simulink model "frame"  (R2020a)
settings: Solver=FixedStepAuto  StartTime=0.0  StopTime=10  FixedStep=1/simVars.freq  RelTol=1e-3
undefined symbols (not defined in the file or in its folder): par, sigbuilder_block, simVars
libraries: simulink x6
settings Model: Creator=Matthias  LastModifiedBy=sihao
settings DataIOCC: ReturnWorkspaceOutputs=off
settings DebuggingCC: ArithmeticOperatorsInVariantConditions=warning
settings SFSimCC: CustomCodeUndefinedFunction=UseInterfaceOnly

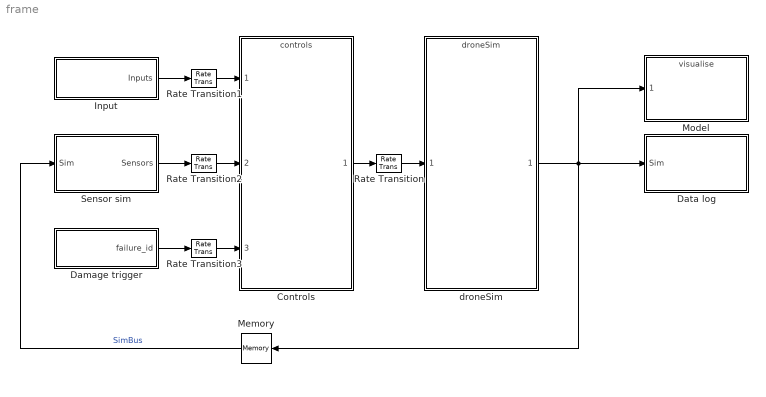
== system frame ==
  Controls : ModelReference  ModelNameDialog=controls  SimulationMode=Normal  ModelReferenceVersion=1.140
  Damage trigger : Subsystem
  Data log : Subsystem
  Input : Subsystem
  Memory : Memory
  Model : ModelReference  ModelNameDialog=visualise.slx  SimulationMode=Normal  ModelReferenceVersion=1.52
  Rate Transition : RateTransition  OutPortSampleTime=1/simVars.freq
  Rate Transition1 : RateTransition  OutPortSampleTime=1/par.freq
  Rate Transition2 : RateTransition  OutPortSampleTime=1/par.freq
  Rate Transition3 : RateTransition  OutPortSampleTime=1/par.freq
  Sensor sim : Subsystem
  droneSim : ModelReference  ModelNameDialog=droneSim  SimulationMode=Normal  ModelReferenceVersion=1.252
  wires:
  Input/1(Inputs) -> Rate Transition1/1
  Sensor sim/1(Sensors) -> Rate Transition2/1
  Memory/1 -> Sensor sim/1(Sim)  "SimBus"
  Rate Transition/1 -> droneSim/1
  Rate Transition1/1 -> Controls/1
  Rate Transition2/1 -> Controls/2
  Controls/1 -> Rate Transition/1
  droneSim/1 -> Model/1, Data log/1(Sim), Memory/1
  Damage trigger/1(failure_id) -> Rate Transition3/1
  Rate Transition3/1 -> Controls/3

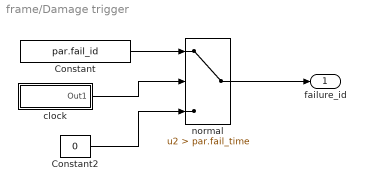
== system frame/Damage trigger ==
  Constant : Constant  Value=par.fail_id
  Constant2 : Constant  Value=0
  clock : Subsystem
  normal : Switch  Criteria=u2 > Threshold  Threshold=par.fail_time
  failure_id : Outport  VectorParamsAs1DForOutWhenUnconnected=off
  wires:
  Constant2/1 -> normal/3
  Constant/1 -> normal/1
  clock/1(Out1) -> normal/2
  normal/1 -> failure_id/1

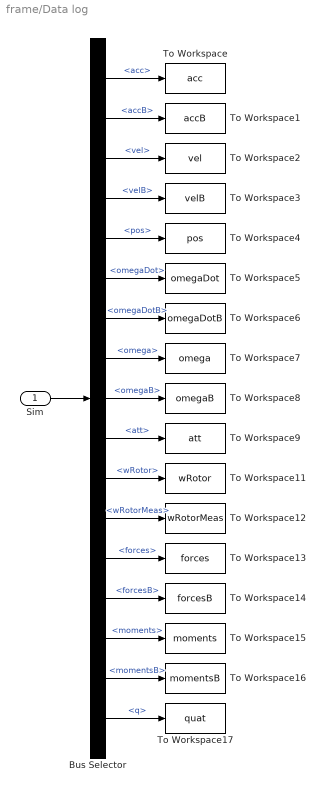
== system frame/Data log ==
  Sim : Inport
  Bus Selector : BusSelector  OutputSignals=acc,accB,vel,velB,pos,omegaDot,omegaDotB,omega,omegaB,att,wRotor,wRotorMeas,forces,forcesB,moments,momentsB,q
  To Workspace : ToWorkspace  VariableName=acc  SaveFormat=Timeseries  SampleTime=-1
  To Workspace1 : ToWorkspace  VariableName=accB  SaveFormat=Timeseries  SampleTime=-1
  To Workspace11 : ToWorkspace  VariableName=wRotor  SaveFormat=Timeseries  SampleTime=-1
  To Workspace12 : ToWorkspace  VariableName=wRotorMeas  SaveFormat=Timeseries  SampleTime=-1
  To Workspace13 : ToWorkspace  VariableName=forces  SaveFormat=Timeseries  SampleTime=-1
  To Workspace14 : ToWorkspace  VariableName=forcesB  SaveFormat=Timeseries  SampleTime=-1
  To Workspace15 : ToWorkspace  VariableName=moments  SaveFormat=Timeseries  SampleTime=-1
  To Workspace16 : ToWorkspace  VariableName=momentsB  SaveFormat=Timeseries  SampleTime=-1
  To Workspace17 : ToWorkspace  VariableName=quat  SaveFormat=Timeseries  SampleTime=-1
  To Workspace2 : ToWorkspace  VariableName=vel  SaveFormat=Timeseries  SampleTime=-1
  To Workspace3 : ToWorkspace  VariableName=velB  SaveFormat=Timeseries  SampleTime=-1
  To Workspace4 : ToWorkspace  VariableName=pos  SaveFormat=Timeseries  SampleTime=-1
  To Workspace5 : ToWorkspace  VariableName=omegaDot  SaveFormat=Timeseries  SampleTime=-1
  To Workspace6 : ToWorkspace  VariableName=omegaDotB  SaveFormat=Timeseries  SampleTime=-1
  To Workspace7 : ToWorkspace  VariableName=omega  SaveFormat=Timeseries  SampleTime=-1
  To Workspace8 : ToWorkspace  VariableName=omegaB  SaveFormat=Timeseries  SampleTime=-1
  To Workspace9 : ToWorkspace  VariableName=att  SaveFormat=Timeseries  SampleTime=-1
  wires:
  Sim/1 -> Bus Selector/1
  Bus Selector/1 -> To Workspace/1  "<acc>"
  Bus Selector/2 -> To Workspace1/1  "<accB>"
  Bus Selector/3 -> To Workspace2/1  "<vel>"
  Bus Selector/4 -> To Workspace3/1  "<velB>"
  Bus Selector/5 -> To Workspace4/1  "<pos>"
  Bus Selector/6 -> To Workspace5/1  "<omegaDot>"
  Bus Selector/7 -> To Workspace6/1  "<omegaDotB>"
  Bus Selector/8 -> To Workspace7/1  "<omega>"
  Bus Selector/9 -> To Workspace8/1  "<omegaB>"
  Bus Selector/10 -> To Workspace9/1  "<att>"
  Bus Selector/11 -> To Workspace11/1  "<wRotor>"
  Bus Selector/12 -> To Workspace12/1  "<wRotorMeas>"
  Bus Selector/13 -> To Workspace13/1  "<forces>"
  Bus Selector/14 -> To Workspace14/1  "<forcesB>"
  Bus Selector/15 -> To Workspace15/1  "<moments>"
  Bus Selector/16 -> To Workspace16/1  "<momentsB>"
  Bus Selector/17 -> To Workspace17/1  "<q>"

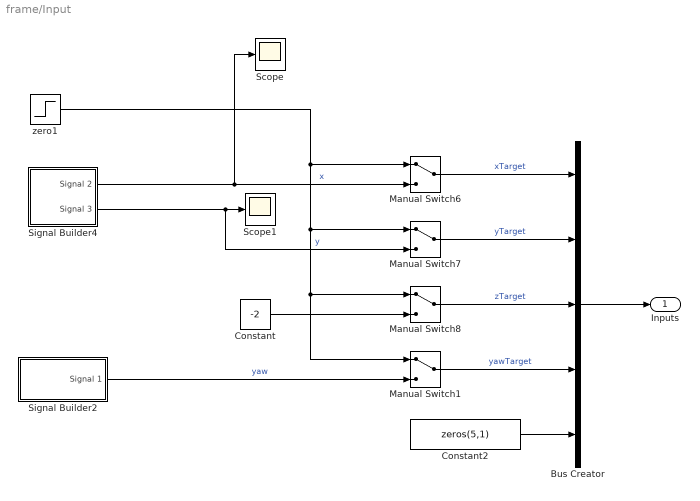
== system frame/Input ==
  Bus Creator : BusCreator  Inputs=5  OutDataTypeStr=Bus: inputsBus
  Constant : Constant  Value=-2
  Constant2 : Constant  Value=zeros(5,1)
  Manual Switch{1,6..8} (4 alike) : ManualSwitch
  Scope : Scope
  Scope1 : Scope
  Signal Builder2 : Subsystem  Tag=STV Subsys  LoadFcn=sigbuilder_block('load');  StartFcn=sigbuilder_block('start');  StopFcn=sigbuilder_block('stop');  ClipboardFcn=sigbuilder_block('clipboard');  mask(Sigbuilder block){tuvar=[0:10]}
      mask help: Simulink:masks:SigbuilderBlock_MD
      mask init:
      | if ~strcmp(get_param(bdroot(gcbh),'SimulationStatus'),'stopped') tuvar = sigbuilder_block('maskInit'); end
      settings: CopyFcn=sigbuilder_block('copy');  DeleteFcn=sigbuilder_block('delete');  ModelCloseFcn=sigbuilder_block('modelClose');  PreSaveFcn=sigbuilder_block('preSave');  PauseFcn=sigbuilder_block('pause');  ContinueFcn=sigbuilder_block('continue');  NameChangeFcn=sigbuilder_block('namechange');  OpenFcn=sigbuilder_block('open',[192.75 285.75 558 394.5 ]);  CloseFcn=sigbuilder_block('close');
      mask Display: plot(0, 0, 100, 100,[2, 2, 32, 32, 2], [68, 8, 8, 68, 68],[32, 2], [38, 38], [32, 19, 2],[53, 60, 44], [32, 17, 17, 2],[16, 16, 31, 31]);txt = getActiveGroup(gcbh);text(2, 100, txt,'verticalAlignment', 'top');
  Signal Builder4 : Subsystem  Tag=STV Subsys  LoadFcn=sigbuilder_block('load',[522.75 156 565.5 354 ]);  StartFcn=sigbuilder_block('start');  StopFcn=sigbuilder_block('stop');  ClipboardFcn=sigbuilder_block('clipboard');  mask(Sigbuilder block){tuvar=[0:10]}
      mask help: Simulink:masks:SigbuilderBlock_MD
      mask init:
      | if ~strcmp(get_param(bdroot(gcbh),'SimulationStatus'),'stopped') tuvar = sigbuilder_block('maskInit'); end
      settings: CopyFcn=sigbuilder_block('copy');  DeleteFcn=sigbuilder_block('delete');  ModelCloseFcn=sigbuilder_block('modelClose');  PreSaveFcn=sigbuilder_block('preSave');  PauseFcn=sigbuilder_block('pause');  ContinueFcn=sigbuilder_block('continue');  NameChangeFcn=sigbuilder_block('namechange');  OpenFcn=sigbuilder_block('open',[526.5 159.75 558 354 ]);  CloseFcn=sigbuilder_block('close');
      mask Display: plot(0, 0, 100, 100,[2, 2, 32, 32, 2], [68, 8, 8, 68, 68],[32, 2], [38, 38], [32, 19, 2],[53, 60, 44], [32, 17, 17, 2],[16, 16, 31, 31]);txt = getActiveGroup(gcbh);text(2, 100, txt,'verticalAlignment', 'top');
  zero1 : Step  Time=3  After=0  SampleTime=0
  Inputs : Outport  OutDataTypeStr=Bus: inputsBus  VectorParamsAs1DForOutWhenUnconnected=off
  wires:
  Bus Creator/1 -> Inputs/1
  Manual Switch1/1 -> Bus Creator/4  "yawTarget"
  Manual Switch8/1 -> Bus Creator/3  "zTarget"
  Constant/1 -> Manual Switch8/2
  Signal Builder4/2(Signal 3) -> Scope1/1, Manual Switch7/2  "y"
  Manual Switch6/1 -> Bus Creator/1  "xTarget"
  Manual Switch7/1 -> Bus Creator/2  "yTarget"
  Signal Builder4/1(Signal 2) -> Scope/1, Manual Switch6/2  "x"
  zero1/1 -> Manual Switch1/1, Manual Switch8/1, Manual Switch7/1, Manual Switch6/1
  Signal Builder2/1(Signal 1) -> Manual Switch1/2  "yaw"
  Constant2/1 -> Bus Creator/5

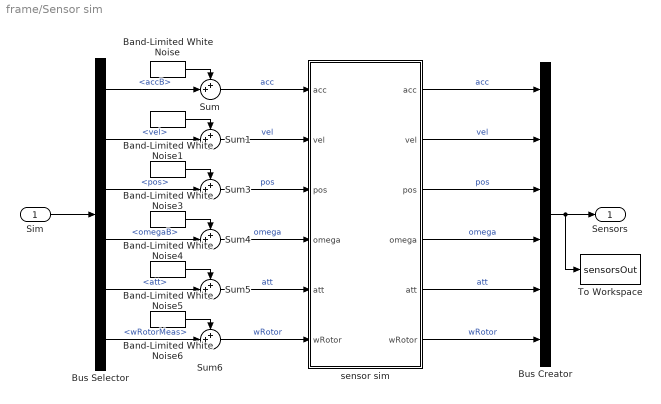
== system frame/Sensor sim ==
  Sim : Inport
  Band-Limited White Noise : simulink/Sources/Band-Limited White Noise  Cov=simVars.sensor.accNoise  Ts=1/par.freq  seed=[23341,23342,23343]
  Band-Limited White Noise1 : simulink/Sources/Band-Limited White Noise  Cov=simVars.sensor.velNoise  Ts=1/par.freq  seed=[23344,23345,23346]
  Band-Limited White Noise3 : simulink/Sources/Band-Limited White Noise  Cov=simVars.sensor.posNoise  Ts=1/par.freq  seed=[23347,23348,23349]
  Band-Limited White Noise4 : simulink/Sources/Band-Limited White Noise  Cov=simVars.sensor.omegaNoise  Ts=1/par.freq  seed=[23350,23351,23352]
  Band-Limited White Noise5 : simulink/Sources/Band-Limited White Noise  Cov=simVars.sensor.attNoise  Ts=1/par.freq  seed=[23353,23354,23355]
  Band-Limited White Noise6 : simulink/Sources/Band-Limited White Noise  Cov=simVars.sensor.wRotorNoise  Ts=1/par.freq  seed=[23356,23357,23358,23359]
  Bus Creator : BusCreator  Inputs=6  OutDataTypeStr=Bus: sensorsBus
      settings: InheritFromInputs=off
  Bus Selector : BusSelector  OutputSignals=accB,vel,pos,omegaB,att,wRotorMeas
  Sum{,1,3..6} (6 alike) : Sum  Inputs=++|
  To Workspace : ToWorkspace  VariableName=sensorsOut  SaveFormat=Timeseries  SampleTime=-1
  sensor sim : MATLAB Function  TreatAsAtomicUnit=on
  Sensors : Outport  OutDataTypeStr=Bus: sensorsBus  VectorParamsAs1DForOutWhenUnconnected=off
  wires:
  Sim/1 -> Bus Selector/1
  Bus Creator/1 -> Sensors/1, To Workspace/1
  Bus Selector/1 -> Sum/2  "<accB>"
  Band-Limited White Noise/1 -> Sum/1
  Bus Selector/2 -> Sum1/2  "<vel>"
  Band-Limited White Noise1/1 -> Sum1/1
  Bus Selector/3 -> Sum3/2  "<pos>"
  Band-Limited White Noise3/1 -> Sum3/1
  Bus Selector/4 -> Sum4/2  "<omegaB>"
  Band-Limited White Noise4/1 -> Sum4/1
  Bus Selector/5 -> Sum5/2  "<att>"
  Band-Limited White Noise5/1 -> Sum5/1
  Bus Selector/6 -> Sum6/2  "<wRotorMeas>"
  Band-Limited White Noise6/1 -> Sum6/1
  Sum/1 -> sensor sim/1("acc ")  "acc"
  Sum1/1 -> sensor sim/2("vel ")  "vel"
  Sum3/1 -> sensor sim/3("pos ")  "pos"
  Sum4/1 -> sensor sim/4("omega ")  "omega"
  Sum5/1 -> sensor sim/5("att ")  "att"
  Sum6/1 -> sensor sim/6("wRotor ")  "wRotor"
  sensor sim/1(acc) -> Bus Creator/1  "acc"
  sensor sim/2(vel) -> Bus Creator/2  "vel"
  sensor sim/3(pos) -> Bus Creator/3  "pos"
  sensor sim/4(omega) -> Bus Creator/4  "omega"
  sensor sim/5(att) -> Bus Creator/5  "att"
  sensor sim/6(wRotor) -> Bus Creator/6  "wRotor"

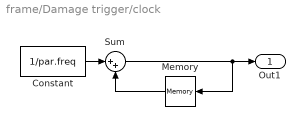
== system frame/Damage trigger/clock ==
  Constant : Constant  Value=1/par.freq
  Memory : Memory
  Sum : Sum  Inputs=|++
  Out1 : Outport  VectorParamsAs1DForOutWhenUnconnected=off
  wires:
  Constant/1 -> Sum/1
  Sum/1 -> Memory/1, Out1/1
  Memory/1 -> Sum/2

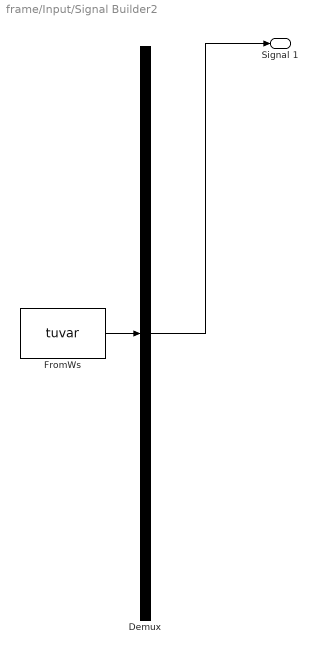
== system frame/Input/Signal Builder2 ==
  Demux : Demux  Tag=STV Demux  Outputs=1
      settings: DisplayOption=none
  FromWs : FromWorkspace  Tag=STV FromWs  VariableName=tuvar
      SigBuilderData=|
      | common.afterFinalStr = 'Extrapolate'
      | common.sampleTime = 0
      | dataSet.timeRange = [0 20]
      | dataSet.name = 'Group 1'
      | sbobj.Groups.Name = 'Group 1'
      | sbobj.Groups.Signals.Name = 'Signal 1'
      | sbobj.Groups.Signals.XData = [0 1.5 20]
      | sbobj.Groups.Signals.YData = [0 3.14 0]
      | sbobj.Groups.TimeRange = [0 20]
  Signal 1 : Outport  Tag=STV Outport  VectorParamsAs1DForOutWhenUnconnected=off
  wires:
  Demux/1 -> Signal 1/1
  FromWs/1 -> Demux/1

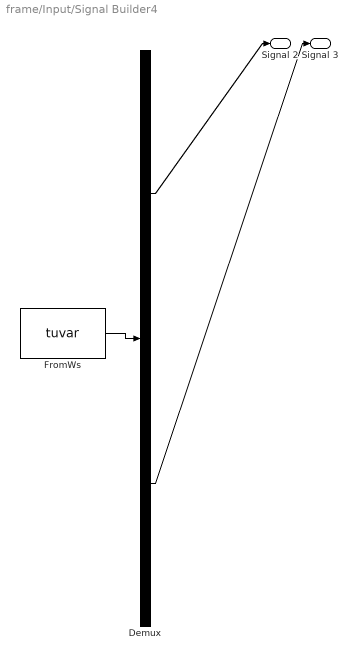
== system frame/Input/Signal Builder4 ==
  Demux : Demux  Tag=STV Demux  Outputs=2
      settings: DisplayOption=none
  FromWs : FromWorkspace  Tag=STV FromWs  VariableName=tuvar
      SigBuilderData=|
      | common.afterFinalStr = 'Extrapolate'
      | common.sampleTime = 0
      | dataSet.timeRange = [0 20]
      | dataSet.name = 'Group 1'
      | sbobj.Groups.Name = 'Group 1'
      | sbobj.Groups.Signals(1).Name = 'Signal 2'
      | sbobj.Groups.Signals(1).XData = [0 1 1 6 6 20]
      | sbobj.Groups.Signals(1).YData = [0 0 3 3 0 0]
      | sbobj.Groups.Signals(2).Name = 'Signal 3'
      | sbobj.Groups.Signals(2).XData = [0 4 4 7.95 7.95 20]
      | sbobj.Groups.Signals(2).YData = [0 0 1.02 1.02 0 0]
      | sbobj.Groups.TimeRange = [0 20]
  Signal 2 : Outport  Tag=STV Outport  VectorParamsAs1DForOutWhenUnconnected=off
  Signal 3 : Outport  Tag=STV Outport  Port=2  VectorParamsAs1DForOutWhenUnconnected=off
  wires:
  Demux/2 -> Signal 3/1
  Demux/1 -> Signal 2/1
  FromWs/1 -> Demux/1

== matlab function frame/Sensor sim/sensor sim ==
  data: acc input; acc output; vel input; pos input; omega input; att input; wRotor input; vel output; pos output; omega output; att output; wRotor output; simVars parameter
function [acc, vel, pos, omega, att, wRotor] = sensorSim(acc, vel, pos, omega, att, wRotor, simVars)

%% add bias to IMU
omega = omega + simVars.sensor.omega_bias';
acc = acc + simVars.sensor.acc_bias';

end
